simulink subsystem "Non_linear_continuous_drone_plant"  (R2020a)
settings: Solver=VariableStepAuto  StartTime=0.0  StopTime=10.0  RelTol=1e-3
settings Model: Creator=augus  LastModifiedBy=augus

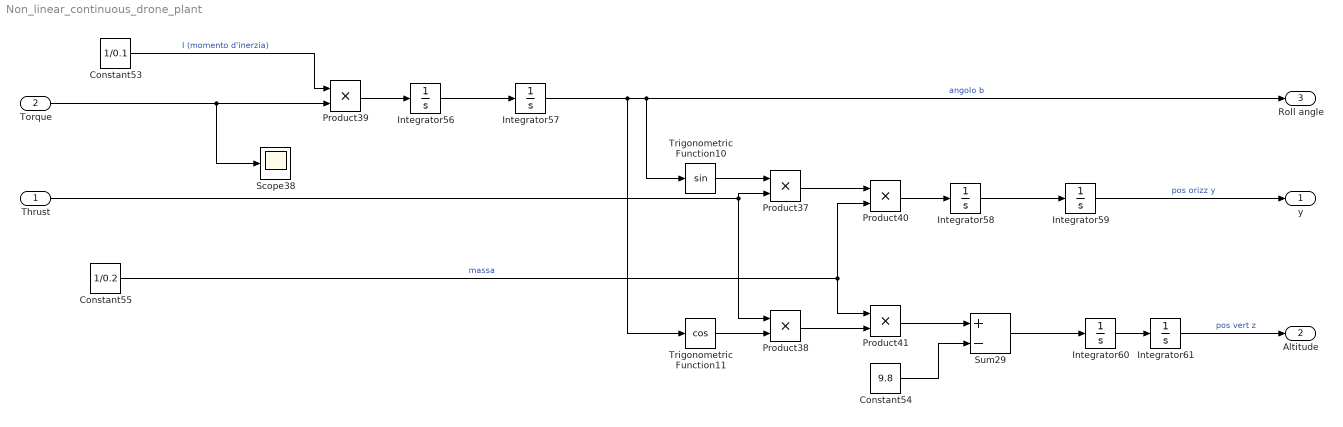
== system Non_linear_continuous_drone_plant ==
  Thrust : Inport  Tag=torque  Description=torque
  Torque : Inport  Tag=thrust  Description=thrust  Port=2
  Constant53 : Constant  Value=1/0.1
  Constant54 : Constant  Value=9.8
  Constant55 : Constant  Value=1/0.2
  Integrator{56..61} (6 alike) : Integrator
  Product{37..41} (5 alike) : Product
  Scope38 : Scope
  Sum29 : Sum  Inputs=+-
  Trigonometric Function10 : Trigonometry
  Trigonometric Function11 : Trigonometry  Operator=cos
  y : Outport  Tag=y position  Description=y position
  Altitude : Outport  Tag=z position  Description=z position  Port=2
  Roll angle : Outport  Tag=roll angle  Description=roll angle  Port=3
  wires:
  Integrator60/1 -> Integrator61/1
  Thrust/1 -> Product37/2, Product38/1
  Sum29/1 -> Integrator60/1
  Integrator56/1 -> Integrator57/1
  Product39/1 -> Integrator56/1
  Torque/1 -> Product39/2, Scope38/1
  Integrator57/1 -> Trigonometric Function10/1, Roll angle/1, Trigonometric Function11/1  "angolo b"
  Product38/1 -> Product41/2
  Constant55/1 -> Product41/1, Product40/2  "massa"
  Product40/1 -> Integrator58/1
  Integrator58/1 -> Integrator59/1
  Product41/1 -> Sum29/1
  Trigonometric Function11/1 -> Product38/2
  Constant54/1 -> Sum29/2
  Trigonometric Function10/1 -> Product37/1
  Product37/1 -> Product40/1
  Integrator61/1 -> Altitude/1  "pos vert z"
  Constant53/1 -> Product39/1  "I (momento d'inerzia)"
  Integrator59/1 -> y/1  "pos orizz y"
